simulink model "Ctrl"  (R2024a)
settings: Solver=FixedStepDiscrete  StartTime=0.0  StopTime=10.0  RelTol=1e-3  EnableMultiTasking=on
settings Model: DataDictionary=dict.sldd  Creator=Administrator  LastModifiedBy=Administrator
settings OptimizationCC: DefaultParameterBehavior=Inlined  EnhancedBackFolding=on  PassReuseOutputArgsAs=Individual arguments  ZeroExternalMemoryAtStartup=off  ZeroInternalMemoryAtStartup=off  OptimizeBlockOrder=speed  DifferentSizesBufferReuse=on  OptimizationCustomize=off  EfficientTunableParamExpr=on
settings DebuggingCC: ParameterTunabilityLossMsg=error
settings SFSimCC: MATLABDynamicMemAlloc=off
settings RTWCC: Description=AUTOSAR  SystemTargetFile=autosar.tlc  GenCodeOnly=on  TemplateMakefile=ert_default_tmf  DataTypeReplacement=CDataTypesFixedWidth
settings CodeAppCC: ForceParamTrailComments=on  IgnoreCustomStorageClasses=off  OperatorAnnotations=on  SimulinkDataObjDesc=on  SFDataObjDesc=on  InsertBlockDesc=on
settings STFCustomTargetCC: MultiwordLength=256  ParMdlRefBuildCompliant=on  CompOptLevelCompliant=on  IncludeMdlTerminateFcn=off  CombineOutputUpdateFcns=on  SuppressErrorStatus=on  ERTCustomFileBanners=on  SupportNonFinite=off  SupportComplex=off  SupportContinuousTime=off  SupportNonInlinedSFcns=off  RemoveResetFunc=on  MATLABClassNameForMDSCustomization=Simulink.SoftwareTarget.ERTCustomization  AutosarCompliant=on  GRTInterface=off  LookupTableObjectStructAxisOrder=2,1,3,4,...  LUTObjectStructOrderEvenSpacing=Size,Table,Breakpoints  SystemTargetFile=autosar.tlc
settings ERTTargetCC: TargetLangStandard=C99 (ISO)  ConcurrentExecutionCompliant=off  IncludeMdlTerminateFcn=off  SuppressErrorStatus=on  SupportNonFinite=off  SupportComplex=off  ModelStepFunctionPrototypeControlCompliant=off  CPPClassGenCompliant=off  AutosarCompliant=on  LookupTableObjectStructAxisOrder=2,1,3,4,...  LUTObjectStructOrderEvenSpacing=Size,Table,Breakpoints  InlinedParameterPlacement=NonHierarchical  ERTCustomFileTemplate=example_file_process.tlc  BooleanTrueId=TRUE  BooleanFalseId=FALSE

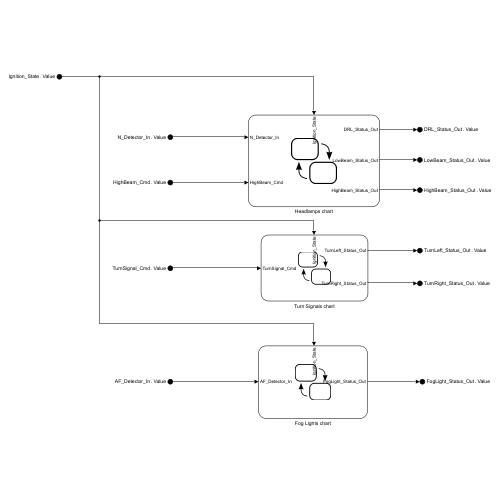
[thumbnail: Simulink's stored preview of the top-level diagram]
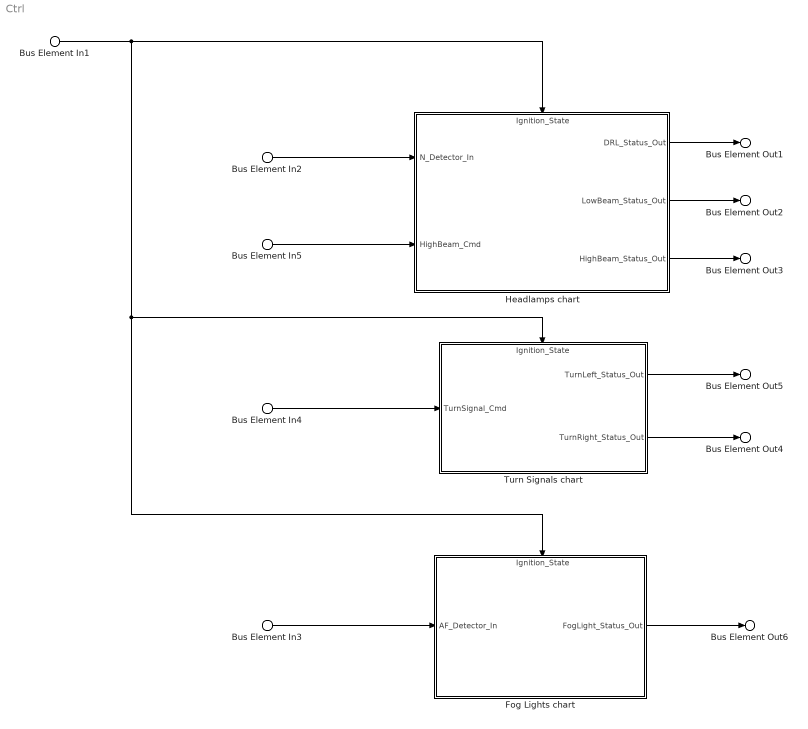
== system Ctrl ==
  Bus Element In2 : Inport  Description=|  PortName=N_Detector_In  Element=Value
      | Sensors detection output values:
      | 0: nothing detected
      | 1: night or fog detected
  Bus Element In3 : Inport  Description=|  Port=2  PortName=AF_Detector_In  Element=Value
      | Sensors detection output values:
      | 0: nothing detected
      | 1: night or fog detected
  Bus Element In5 : Inport  Description=|  Port=3  PortName=HighBeam_Cmd  Element=Value
      | User command for high Beam activation
      | 0: OFF
      | 1: ON
  Bus Element In4 : Inport  Port=4  PortName=TurnSignal_Cmd  Element=Value
  Bus Element In1 : Inport  Description=|  Port=5  PortName=Ignition_State  Element=Value
      | Ignition State:
      | 0: OFF
      | 1: ON
  Fog Lights chart : Stateflow chart  TreatAsAtomicUnit=on
      settings: PortSchema="{\"entries\":[{\"content\":{\"sides\":[{\"content\":{\"connectorIds\":[\"In1\"]},\"type\":\"ConnectorPlacement.EquallySpacedRectSide\",\"uuid\":\"6e73d07d-318a-4fa0-9ed3-6e487adbbe97\"},{\"content\":{\"connectorIds\":[\"Out1\"],\"side\":\"RIGHT\"},\"type\":\"ConnectorPlacement.EquallySpacedRectSide\",\"uuid\":\"c78fcebb-7682-40eb-b9d7-f57ee830b124\"},{\"content\":{\"connectorIds\":[\"In2\"],\"side\":\"TOP\"},\"type\":\"ConnectorPlacement.EquallySpacedRectSide\",\"uuid\":\"a46668cb-eeb1-4573-b012-4867c50e75e2\"}]},\"type\":\"ConnectorPlacement.EquallySpacedConnector\",\"uuid\":\"9a4e117f-bbac-4ba4-b023-05aa8e8d359e\"}],\"packageUris\":[\"http://schema.mathworks.com/mf0/Connector/R2020b\"],\"version\":\"1.0\"}"
  Headlamps chart : Stateflow chart  TreatAsAtomicUnit=on
      settings: PortSchema="{\"entries\":[{\"content\":{\"sides\":[{\"content\":{\"connectorIds\":[\"In2\",\"In3\"]},\"type\":\"ConnectorPlacement.EquallySpacedRectSide\",\"uuid\":\"9fe301b6-896c-4ff4-90e3-e98f5e2eb580\"},{\"content\":{\"connectorIds\":[\"Out1\",\"Out2\",\"Out3\"],\"side\":\"RIGHT\"},\"type\":\"ConnectorPlacement.EquallySpacedRectSide\",\"uuid\":\"5681ff8b-5b1b-4a6b-9ff5-476e06331b1c\"},{\"content\":{\"connectorIds\":[\"In1\"],\"side\":\"TOP\"},\"type\":\"ConnectorPlacement.EquallySpacedRectSide\",\"uuid\":\"a316b609-19d8-4a99-b7c9-86636a53fc41\"}]},\"type\":\"ConnectorPlacement.EquallySpacedConnector\",\"uuid\":\"451f7b41-3bcf-4e28-af12-1efa4b6b4571\"}],\"packageUris\":[\"http://schema.mathworks.com/mf0/Connector/R2020b\"],\"version\":\"1.0\"}"
  Turn Signals chart : Stateflow chart  TreatAsAtomicUnit=on
      settings: PortSchema="{\"entries\":[{\"content\":{\"sides\":[{\"content\":{\"connectorIds\":[\"In2\"]},\"type\":\"ConnectorPlacement.EquallySpacedRectSide\",\"uuid\":\"21e077f9-b9df-45da-8d86-5a77e5896ec7\"},{\"content\":{\"connectorIds\":[\"Out1\",\"Out2\"],\"side\":\"RIGHT\"},\"type\":\"ConnectorPlacement.EquallySpacedRectSide\",\"uuid\":\"d233b554-accc-4876-a8f7-7abcf56a3c72\"},{\"content\":{\"connectorIds\":[\"In1\"],\"side\":\"TOP\"},\"type\":\"ConnectorPlacement.EquallySpacedRectSide\",\"uuid\":\"b1f6256c-b5f1-4198-aca6-dbe9e4529c01\"}]},\"type\":\"ConnectorPlacement.EquallySpacedConnector\",\"uuid\":\"06e2a0ae-4dc1-432c-926b-d55e6c3016e0\"}],\"packageUris\":[\"http://schema.mathworks.com/mf0/Connector/R2020b\"],\"version\":\"1.0\"}"
  Bus Element Out1 : Outport  Description=|  PortName=DRL_Status_Out  Element=Value
      | Lights state On or OFF (LowBeam, HighBeam, DRL, FogLight, ...):
      | 0: Light should be OFF
      | 1: Light should be ON
  Bus Element Out2 : Outport  Description=|  Port=2  PortName=LowBeam_Status_Out  Element=Value
      | Lights state On or OFF (LowBeam, HighBeam, DRL, FogLight, ...):
      | 0: Light should be OFF
      | 1: Light should be ON
  Bus Element Out3 : Outport  Description=|  Port=3  PortName=HighBeam_Status_Out  Element=Value
      | Lights state On or OFF (LowBeam, HighBeam, DRL, FogLight, ...):
      | 0: Light should be OFF
      | 1: Light should be ON
  Bus Element Out4 : Outport  Description=|  Port=4  PortName=TurnRight_Status_Out  Element=Value
      | Lights state On or OFF (LowBeam, HighBeam, DRL, FogLight, ...):
      | 0: Light should be OFF
      | 1: Light should be ON
  Bus Element Out5 : Outport  Description=|  Port=5  PortName=TurnLeft_Status_Out  Element=Value
      | Lights state On or OFF (LowBeam, HighBeam, DRL, FogLight, ...):
      | 0: Light should be OFF
      | 1: Light should be ON
  Bus Element Out6 : Outport  Description=|  Port=6  PortName=FogLight_Status_Out  Element=Value
      | Lights state On or OFF (LowBeam, HighBeam, DRL, FogLight, ...):
      | 0: Light should be OFF
      | 1: Light should be ON
  wires:
  Headlamps chart/3(HighBeam_Status_Out) -> Bus Element Out3/1
  Bus Element In2/1 -> Headlamps chart/2(N_Detector_In)
  Turn Signals chart/1(TurnLeft_Status_Out) -> Bus Element Out5/1
  Bus Element In4/1 -> Turn Signals chart/2(TurnSignal_Cmd)
  Turn Signals chart/2(TurnRight_Status_Out) -> Bus Element Out4/1
  Bus Element In3/1 -> Fog Lights chart/1(AF_Detector_In)
  Fog Lights chart/1(FogLight_Status_Out) -> Bus Element Out6/1
  Bus Element In5/1 -> Headlamps chart/3(HighBeam_Cmd)
  Headlamps chart/1(DRL_Status_Out) -> Bus Element Out1/1
  Bus Element In1/1 -> Headlamps chart/1(Ignition_State), Turn Signals chart/1(Ignition_State), Fog Lights chart/2(Ignition_State)
  Headlamps chart/2(LowBeam_Status_Out) -> Bus Element Out2/1

== stateflow chart Ctrl/Turn Signals chart ==
  settings: updateMethod=DISCRETE  sampleTime=2  executeAtInitialization=1  initializeOutput=1
  state Blink_State1
    entry:
    TurnLeft_Status_Out = ~TurnLeft_Status_Out;
  state Blink_State
    entry:
    TurnRight_Status_Out = ~TurnRight_Status_Out;
  state TurnLeft_Active_State
    entry:
    TurnLeft_Status_Out = true;
    TurnRight_Status_Out = false;
  state TurnRight_Active_State
    entry:
    TurnLeft_Status_Out = false;
    TurnRight_Status_Out = true;
  state TurnLights_Idle_State
    entry:
    TurnRight_Status_Out = false;
    TurnLeft_Status_Out = false;
  Blink_State -> Blink_State1 [order 3] : [TurnSignal_Cmd == 2]
  Blink_State1 -> Blink_State [order 3] : [TurnSignal_Cmd == 1]
  Blink_State -> TurnLights_Idle_State [order 2] : [Ignition_State == 0]
  Blink_State1 -> TurnLights_Idle_State [order 1] : [Ignition_State == 0]
  Blink_State1 -> TurnLeft_Active_State [order 2] : [after(2, tick)]
  TurnLeft_Active_State -> Blink_State1 [order 2] : [after(2, tick)]
  TurnRight_Active_State -> Blink_State [order 2] : [after(2, tick)]
  Blink_State -> TurnRight_Active_State [order 1] : [after(2, tick)]
  (default) -> TurnLights_Idle_State
  TurnLights_Idle_State -> TurnLeft_Active_State [order 2] : [Ignition_State == 1 && TurnSignal_Cmd == 2]
  TurnLights_Idle_State -> TurnRight_Active_State [order 1] : [Ignition_State == 1 && TurnSignal_Cmd == 1]
  TurnLeft_Active_State -> TurnLights_Idle_State [order 1] : [Ignition_State == 1 && TurnSignal_Cmd ==  0]
  TurnRight_Active_State -> TurnLights_Idle_State [order 1] : [Ignition_State == 1 && TurnSignal_Cmd == 0]
  TurnLights_Idle_State -> TurnLights_Idle_State [order 3] : [Ignition_State == 0]
  data: Ignition_State input; TurnSignal_Cmd input; TurnLeft_Status_Out output; TurnRight_Status_Out output

== stateflow chart Ctrl/Fog Lights chart ==
  settings: updateMethod=DISCRETE  sampleTime=2  executeAtInitialization=1  initializeOutput=1
  state Idle_State
    entry:
    FogLight_Status_Out = false;
  state FogLight_Active_State
    entry:
    FogLight_Status_Out = true;
  (default) -> Idle_State
  FogLight_Active_State -> Idle_State : [Ignition_State == 0 || AF_Detector_In == 0]
  Idle_State -> FogLight_Active_State [order 2] : [Ignition_State == 1 && AF_Detector_In == 1]
  Idle_State -> Idle_State [order 1] : [Ignition_State == 0]
  data: AF_Detector_In input; FogLight_Status_Out output; Ignition_State input

== stateflow chart Ctrl/Headlamps chart ==
  settings: updateMethod=DISCRETE  sampleTime=2  executeAtInitialization=1  initializeOutput=1
  state Lighting_Level
    state DayRunningLights_Active_State
      entry:
      DRL_Status_Out = 1;
      LowBeam_Status_Out = 0;
      HighBeam_Status_Out = 0;
    state LowBeam_Active_State
      entry:
      DRL_Status_Out = 0;
      LowBeam_Status_Out = 1;
      HighBeam_Status_Out = 0;
    state HighBeam_Active_State
      entry:
      LowBeam_Status_Out = 0;
      HighBeam_Status_Out = 1;
    (default) -> DayRunningLights_Active_State
    DayRunningLights_Active_State -> LowBeam_Active_State : [N_Detector_In == 1]
    LowBeam_Active_State -> DayRunningLights_Active_State [order 2] : [N_Detector_In != 1]
    LowBeam_Active_State -> HighBeam_Active_State [order 1] : [HighBeam_Cmd == 1]
    HighBeam_Active_State -> LowBeam_Active_State [order 1] : [HighBeam_Cmd != 1]
    HighBeam_Active_State -> DayRunningLights_Active_State [order 2] : [N_Detector_In != 1]
  state Idle_State
    entry:
    DRL_Status_Out = 0;
    LowBeam_Status_Out = 0;
    HighBeam_Status_Out = 0;
  (default) -> Idle_State
  Idle_State -> Lighting_Level [order 2] : [Ignition_State == 1]
  Lighting_Level -> Idle_State : [Ignition_State != 1]
  Idle_State -> Idle_State [order 1] : [Ignition_State == 0]
  data: Ignition_State input; N_Detector_In input; HighBeam_Cmd input; DRL_Status_Out output; LowBeam_Status_Out output; HighBeam_Status_Out output
